simulink model "model5"  (R2023a)
settings: Solver=VariableStepAuto  StartTime=0.0  StopTime=40  RelTol=1e-3
settings Model: Creator=evdokiiagalkina  LastModifiedBy=evdokiiagalkina

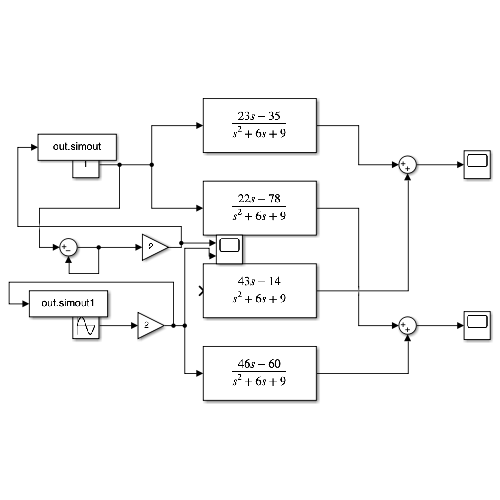
[thumbnail: Simulink's stored preview of the top-level diagram]
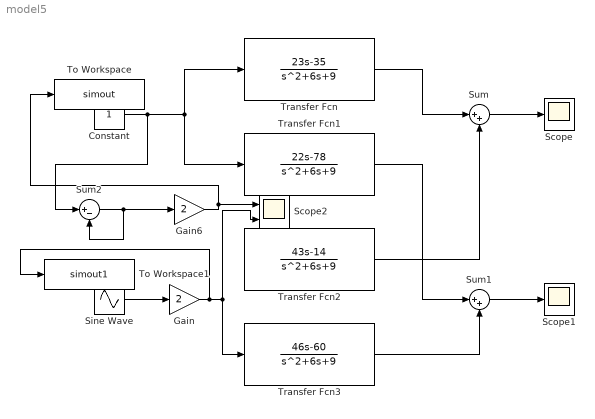
== system model5 ==
  Constant : Constant
  Gain : Gain  Gain=2
  Gain6 : Gain  Gain=2
  Scope : Scope
  Scope1 : Scope
  Scope2 : Scope  NumInputPorts=2
  Sine Wave : Sin  SampleTime=0
  Sum : Sum  Inputs=|++
  Sum1 : Sum  Inputs=|++
  Sum2 : Sum  Inputs=|+-
  To Workspace : ToWorkspace  VariableName=simout  SaveFormat=Timeseries  SampleTime=-1
  To Workspace1 : ToWorkspace  VariableName=simout1  SaveFormat=Timeseries  SampleTime=-1
  Transfer Fcn : TransferFcn  Numerator=[23,-35]  Denominator=[1,6,9]
  Transfer Fcn1 : TransferFcn  Numerator=[22,-78]  Denominator=[1,6,9]
  Transfer Fcn2 : TransferFcn  Numerator=[43,-14]  Denominator=[1,6,9]
  Transfer Fcn3 : TransferFcn  Numerator=[46,-60]  Denominator=[1,6,9]
  wires:
  Sine Wave/1 -> Gain/1
  Transfer Fcn/1 -> Sum/1
  Transfer Fcn2/1 -> Sum/2
  Transfer Fcn1/1 -> Sum1/1
  Transfer Fcn3/1 -> Sum1/2
  Sum1/1 -> Scope1/1
  Sum/1 -> Scope/1
  Sum2/1 -> Gain6/1, Sum2/2
  Constant/1 -> Sum2/1, Transfer Fcn1/1, Transfer Fcn/1
  Gain6/1 -> To Workspace/1, Scope2/1
  Gain/1 -> To Workspace1/1, Scope2/2, Transfer Fcn3/1
